simulink model "sinavsoru2"  (R2023b)
settings: Solver=VariableStepAuto  StartTime=0.0  StopTime=10.0  RelTol=1e-3
settings Model: Creator=yasinsensoy  LastModifiedBy=yasinsensoy

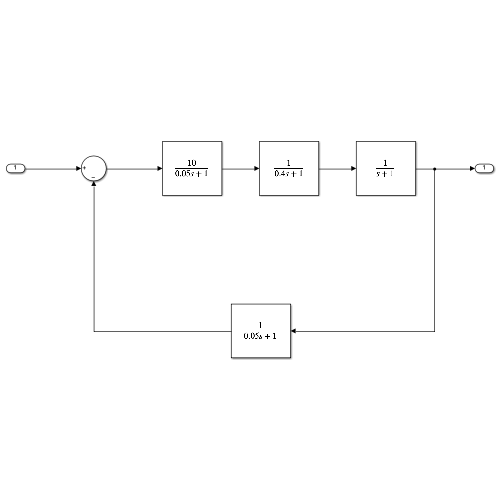
[thumbnail: Simulink's stored preview of the top-level diagram]
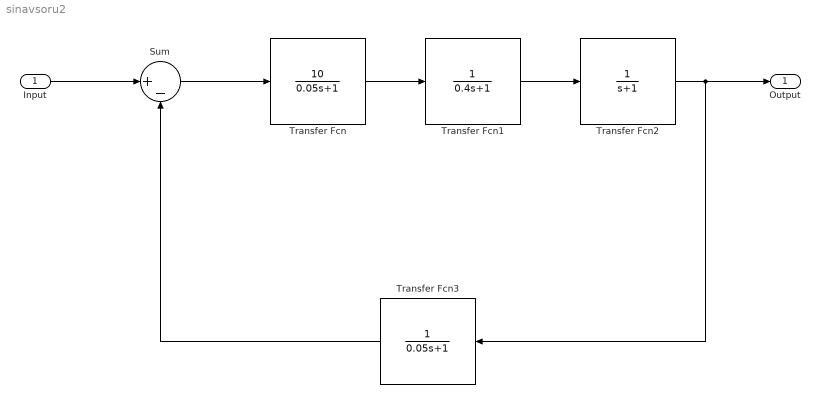
== system sinavsoru2 ==
  Input : Inport
  Sum : Sum  Inputs=|+-
  Transfer Fcn : TransferFcn  Numerator=[10]  Denominator=[0.05 1]
  Transfer Fcn1 : TransferFcn  Denominator=[0.4 1]
  Transfer Fcn2 : TransferFcn  Denominator=[1 1]
  Transfer Fcn3 : TransferFcn  Denominator=[0.05 1]
  Output : Outport
  wires:
  Transfer Fcn3/1 -> Sum/2
  Sum/1 -> Transfer Fcn/1
  Transfer Fcn/1 -> Transfer Fcn1/1
  Transfer Fcn1/1 -> Transfer Fcn2/1
  Transfer Fcn2/1 -> Output/1, Transfer Fcn3/1
  Input/1 -> Sum/1
